simulink model "instalatie_cu_filtru"  (R2022b)
settings: Solver=VariableStepAuto  StartTime=0.0  StopTime=10.0  RelTol=1e-3
values from neighbouring files (symbols this model uses):
  k = 0.035    [date_indrumator.m]    (also in proiect.m)
  k11 = k2^2 + 4*(k - k3)*k1    (= 0.08909684)    [date_indrumator.m]    (also in proiect.m = 0.08885985)
  k12 = 8*(k-k3)    (= 0.2848)    [date_indrumator.m]    (also in proiect.m)
  k13 = 2*(k-k3)    (= 0.0712)    [date_indrumator.m]    (also in proiect.m)
  k2 = -0.015    [date_indrumator.m]    (also in proiect.m = -0.0015)
  keta = 8*(10^-5)    (= 8e-05)    [date_indrumator.m]    (also in proiect.m)
settings Model: Creator=Ruxandra  LastModifiedBy=Ruxandra

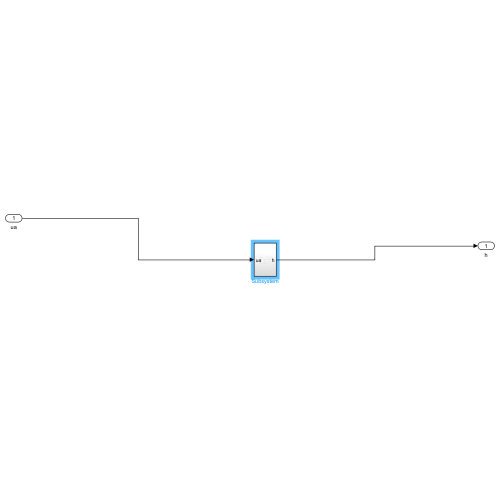
[thumbnail: Simulink's stored preview of the top-level diagram]
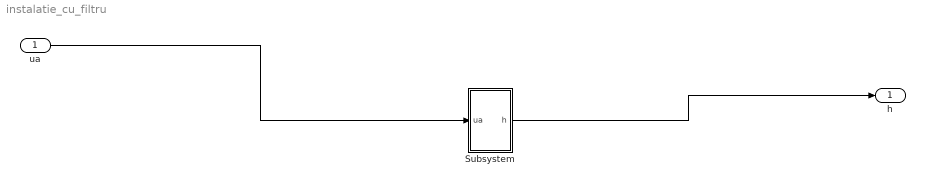
== system instalatie_cu_filtru ==
  ua : Inport
  Subsystem : Subsystem
  h : Outport
  wires:
  ua/1 -> Subsystem/1(ua)
  Subsystem/1(h) -> h/1

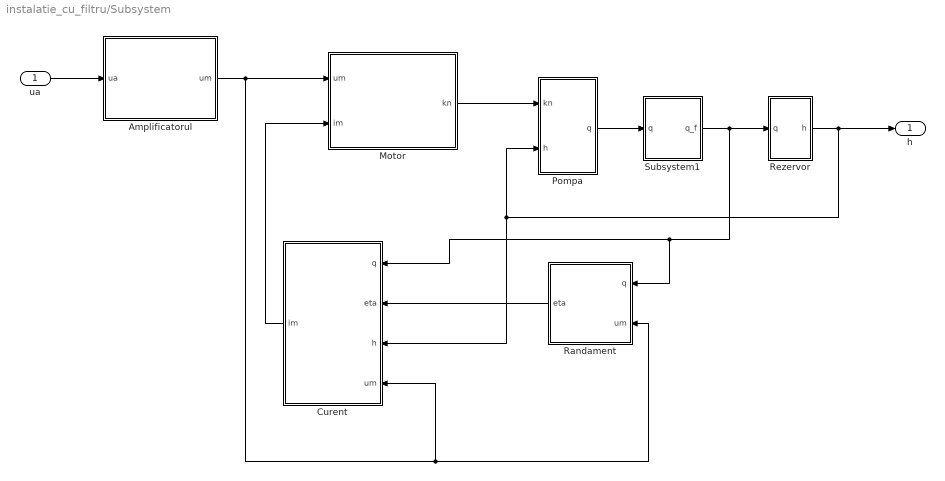
== system instalatie_cu_filtru/Subsystem ==
  ua : Inport
  Amplificatorul : Subsystem
  Curent : Subsystem
  Motor : Subsystem
  Pompa : Subsystem
  Randament : Subsystem
  Rezervor : Subsystem
  Subsystem1 : Subsystem
  h : Outport
  wires:
  Amplificatorul/1(um) -> Motor/1(um), Curent/4(um), Randament/2(um)
  Rezervor/1(h) -> h/1, Pompa/2(h), Curent/3(h)
  Motor/1("kn ") -> Pompa/1(kn)
  ua/1 -> Amplificatorul/1(ua)
  Randament/1(eta) -> Curent/2(eta)
  Curent/1(im) -> Motor/2(im)
  Subsystem1/1(q_f) -> Rezervor/1(q), Curent/1(q), Randament/1(q)
  Pompa/1(q) -> Subsystem1/1(q)

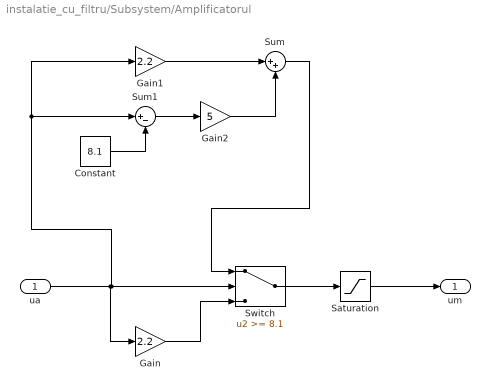
== system instalatie_cu_filtru/Subsystem/Amplificatorul ==
  ua : Inport
  Constant : Constant  Value=8.1
  Gain : Gain  Gain=2.2
  Gain1 : Gain  Gain=2.2
  Gain2 : Gain  Gain=5
  Saturation : Saturate  UpperLimit=22  LowerLimit=0
  Sum : Sum  Inputs=|++
  Sum1 : Sum  Inputs=|+-
  Switch : Switch  Threshold=8.1  RndMeth=Nearest  SaturateOnIntegerOverflow=off  InputSameDT=off
  um : Outport
  wires:
  Gain1/1 -> Sum/1
  ua/1 -> Sum1/1, Gain1/1, Switch/2, Gain/1
  Saturation/1 -> um/1
  Gain/1 -> Switch/3
  Gain2/1 -> Sum/2
  Sum1/1 -> Gain2/1
  Sum/1 -> Switch/1
  Switch/1 -> Saturation/1
  Constant/1 -> Sum1/2

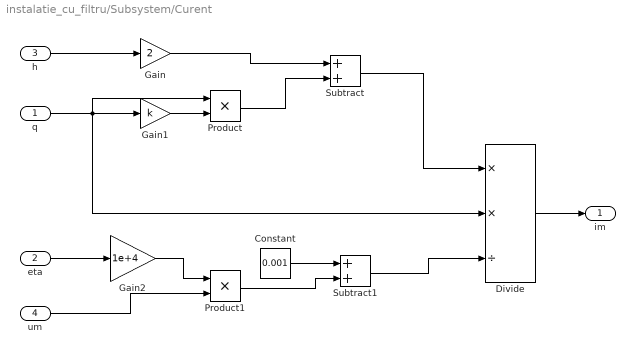
== system instalatie_cu_filtru/Subsystem/Curent ==
  q : Inport
  eta : Inport  Port=2
  h : Inport  Port=3
  um : Inport  Port=4
  Constant : Constant  Value=0.001
  Divide : Product  Inputs=**/
  Gain : Gain  Gain=2
  Gain1 : Gain  Gain=k
  Gain2 : Gain  Gain=1e+4
  Product : Product
  Product1 : Product
  Subtract : Sum
  Subtract1 : Sum
  im : Outport
  wires:
  Product/1 -> Subtract/2
  h/1 -> Gain/1
  Gain/1 -> Subtract/1
  Subtract1/1 -> Divide/3
  Gain2/1 -> Product1/1
  Constant/1 -> Subtract1/1
  Subtract/1 -> Divide/1
  Gain1/1 -> Product/2
  eta/1 -> Gain2/1
  Product1/1 -> Subtract1/2
  q/1 -> Divide/2, Gain1/1, Product/1
  um/1 -> Product1/2
  Divide/1 -> im/1

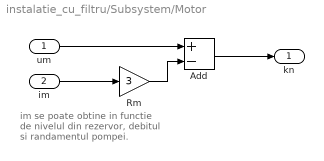
== system instalatie_cu_filtru/Subsystem/Motor ==
  note: im se poate obtine in functie de nivelul din rezervor, debitul si randamentul pompei.
  um : Inport
  im : Inport  Port=2
  Add : Sum  Inputs=+-
  Rm : Gain  Gain=3
  "kn " : Outport
  wires:
  im/1 -> Rm/1
  um/1 -> Add/1
  Rm/1 -> Add/2
  Add/1 -> "kn "/1

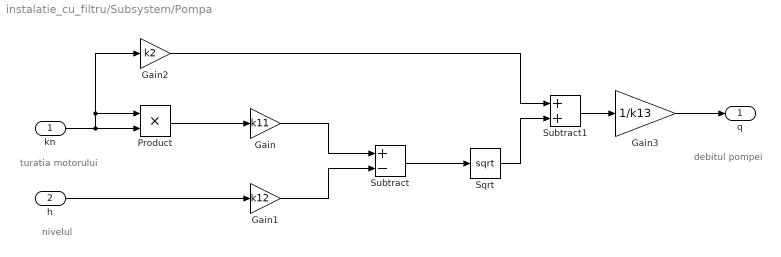
== system instalatie_cu_filtru/Subsystem/Pompa ==
  note: debitul pompei
  note: nivelul
  note: turatia motorului
  kn : Inport
  h : Inport  Port=2
  Gain : Gain  Gain=k11
  Gain1 : Gain  Gain=k12
  Gain2 : Gain  Gain=k2
  Gain3 : Gain  Gain=1/k13
  Product : Product
  Sqrt : Sqrt
  Subtract : Sum  Inputs=+-
  Subtract1 : Sum
  q : Outport
  wires:
  Sqrt/1 -> Subtract1/2
  Gain1/1 -> Subtract/2
  h/1 -> Gain1/1
  Gain2/1 -> Subtract1/1
  kn/1 -> Product/1, Gain2/1, Product/2
  Subtract/1 -> Sqrt/1
  Subtract1/1 -> Gain3/1
  Gain/1 -> Subtract/1
  Gain3/1 -> q/1
  Product/1 -> Gain/1

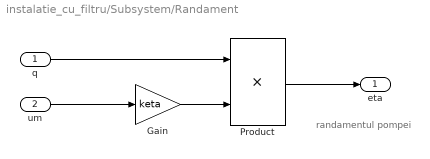
== system instalatie_cu_filtru/Subsystem/Randament ==
  note: randamentul pompei
  q : Inport
  um : Inport  Port=2
  Gain : Gain  Gain=keta
  Product : Product
  eta : Outport
  wires:
  um/1 -> Gain/1
  Product/1 -> eta/1
  q/1 -> Product/1
  Gain/1 -> Product/2

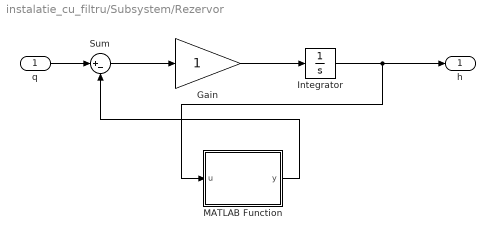
== system instalatie_cu_filtru/Subsystem/Rezervor ==
  q : Inport
  Gain : Gain
  Integrator : Integrator
  MATLAB Function : MATLAB Function  TreatAsAtomicUnit=on
  Sum : Sum  Inputs=|+-
  h : Outport
  wires:
  Integrator/1 -> h/1, MATLAB Function/1(u)
  q/1 -> Sum/1
  Gain/1 -> Integrator/1
  MATLAB Function/1(y) -> Sum/2
  Sum/1 -> Gain/1

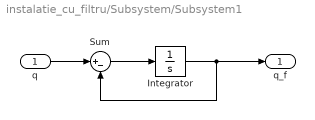
== system instalatie_cu_filtru/Subsystem/Subsystem1 ==
  q : Inport
  Integrator : Integrator
  Sum : Sum  Inputs=|+-
  q_f : Outport
  wires:
  q/1 -> Sum/1
  Integrator/1 -> q_f/1, Sum/2
  Sum/1 -> Integrator/1

== matlab function instalatie_cu_filtru/Subsystem/Rezervor/MATLAB Function ==
  data: u input; y output
function y = sqrt(u)

y = sqrt(u)*9;
